simulink model "car_following"  (R2016b)
settings: Solver=FixedStepAuto  StartTime=0.0  StopTime=20  FixedStep=0.1  RelTol=1e-3
libraries: simulink x1
settings Model: Creator=boran  LastModifiedBy=boran

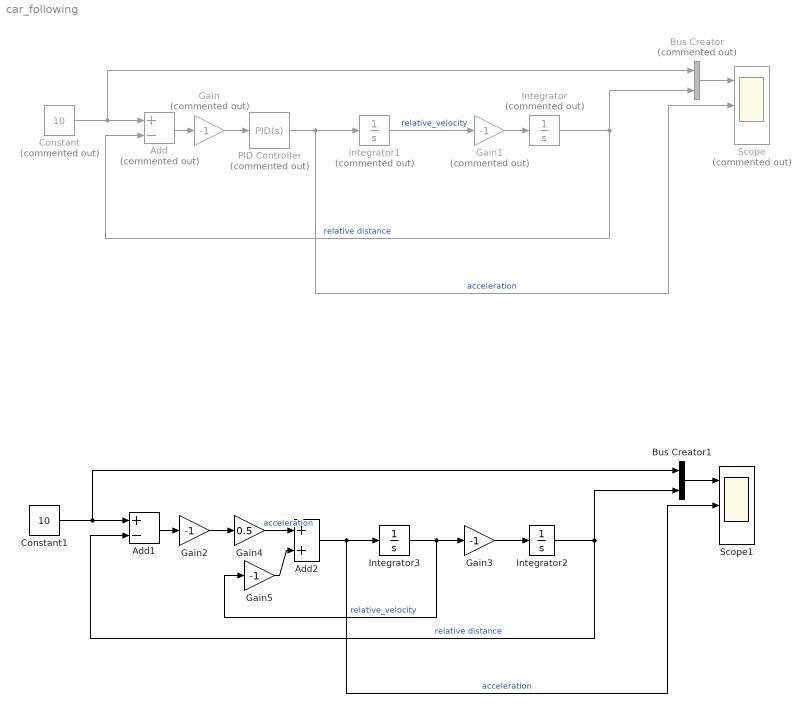
== system car_following ==
  Add : Sum  Commented=on  Inputs=+-
  Add1 : Sum  Inputs=+-
  Add2 : Sum
  Bus Creator : BusCreator  Commented=on  Inputs=2
  Bus Creator1 : BusCreator  Inputs=2
  Constant : Constant  Commented=on  Value=10
  Constant1 : Constant  Value=10
  Gain : Gain  Commented=on  Gain=-1
  Gain1 : Gain  Commented=on  Gain=-1
  Gain2 : Gain  Gain=-1
  Gain3 : Gain  Gain=-1
  Gain4 : Gain  Gain=0.5
  Gain5 : Gain  Gain=-1
  Integrator : Integrator  Commented=on  InitialCondition=15
  Integrator1 : Integrator  Commented=on
  Integrator2 : Integrator  InitialCondition=15
  Integrator3 : Integrator
  PID Controller : simulink/Continuous/PID Controller  Commented=on  Controller=PID  TimeDomain=Continuous-time  SampleTime=-1  IntegratorMethod=Forward Euler  FilterMethod=Forward Euler  Form=Parallel  UseFilter=on  ControllerParametersSource=internal  P=0.5  I=0  D=1  N=10000  InitialConditionSource=internal  InitialConditionForIntegrator=0  InitialConditionForFilter=0  ExternalReset=none  LimitOutput=on  UpperSaturationLimit=9.8  LowerSaturationLimit=-9.8*0.9  LinearizeAsGain=on  AntiWindupMode=none  Kb=1  TrackingMode=off  Kt=1  PParamMin=[]  PParamMax=[]  IParamMin=[]  IParamMax=[]  DParamMin=[]  DParamMax=[]  NParamMin=[]  NParamMax=[]  KbParamMin=[]  KbParamMax=[]  KtParamMin=[]  KtParamMax=[]  POutMin=[]  POutMax=[]  IOutMin=[]  IOutMax=[]  DOutMin=[]  DOutMax=[]  NOutMin=[]  NOutMax=[]  KbOutMin=[]  KbOutMax=[]  KtOutMin=[]  KtOutMax=[]  IntegratorOutMin=[]  IntegratorOutMax=[]  FilterOutMin=[]  FilterOutMax=[]  SumOutMin=[]  SumOutMax=[]  SumI1OutMin=[]  SumI1OutMax=[]  SumI2OutMin=[]  SumI2OutMax=[]  SumI3OutMin=[]  SumI3OutMax=[]  SumDOutMin=[]  SumDOutMax=[]  SaturationOutMin=[]  SaturationOutMax=[]  IntegratorContinuousStateAttributes=''  IntegratorStateMustResolveToSignalObject=off  IntegratorRTWStateStorageClass=Auto  FilterContinuousStateAttributes=''  FilterStateMustResolveToSignalObject=off  FilterRTWStateStorageClass=Auto  DifferentiatorICPrevScaledInput=0  DifferentiatorOutMin=[]  DifferentiatorOutMax=[]
  Scope : Scope  Commented=on  NumInputPorts=3
  Scope1 : Scope  NumInputPorts=3
  wires:
  Add/1 -> Gain/1
  Integrator/1 -> Add/2, Bus Creator/2  "relative distance"
  PID Controller/1 -> Integrator1/1, Scope/2  "acceleration"
  Integrator1/1 -> Gain1/1  "relative_velocity"
  Bus Creator/1 -> Scope/1
  Constant/1 -> Bus Creator/1, Add/1
  Gain/1 -> PID Controller/1
  Gain1/1 -> Integrator/1
  Add1/1 -> Gain2/1
  Integrator2/1 -> Add1/2, Bus Creator1/2  "relative distance"
  Add2/1 -> Scope1/2, Integrator3/1  "acceleration"
  Integrator3/1 -> Gain5/1, Gain3/1  "relative_velocity"
  Bus Creator1/1 -> Scope1/1
  Constant1/1 -> Bus Creator1/1, Add1/1
  Gain2/1 -> Gain4/1
  Gain3/1 -> Integrator2/1
  Gain4/1 -> Add2/1  "acceleration"
  Gain5/1 -> Add2/2
